simulink model "SistemaLabo_2023a"  (R2024b)
settings: Solver=VariableStepAuto  StartTime=0.0  StopTime=100  MaxStep=1e-2  RelTol=1e-3
libraries: slident x1
settings Model: Creator=david
settings DebuggingCC: UnconnectedInputMsg=warning  UnconnectedOutputMsg=warning  UnconnectedLineMsg=warning
settings ModelReferenceCC: EnableRefExpFcnMdlSchedulingChecks=on
settings RTWCC: GPUComputeCapability=3.5  DLArmComputeVersion=19.05

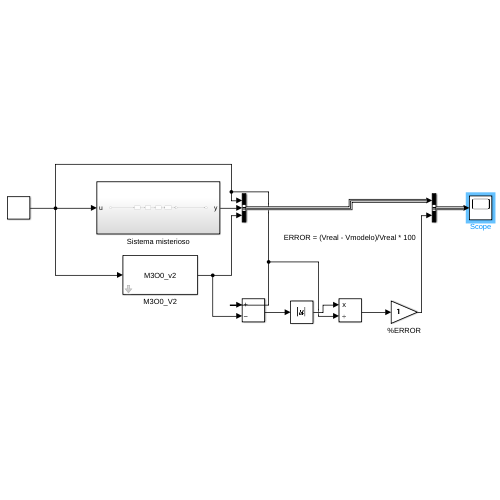
[thumbnail: Simulink's stored preview of the top-level diagram]
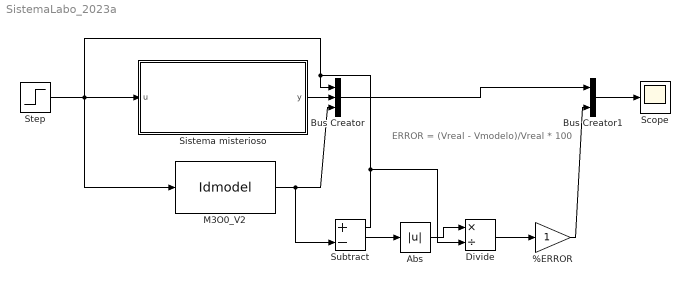
== system SistemaLabo_2023a ==
  note: ERROR = (Vreal - Vmodelo)/Vreal * 100
  %ERROR : Gain
  Abs : Abs  SaturateOnIntegerOverflow=off
  Bus Creator : BusCreator  Inputs=3
  Bus Creator1 : BusCreator  Inputs=2
  Divide : Product  Inputs=*/
  M3O0_V2 : slident/Models/Idmodel  sys=M3O0_v2  IC=0  noi=on  seed=[]
  Scope : Scope
  Sistema misterioso : Subsystem
  Step : Step  SampleTime=0
  Subtract : Sum  Inputs=+-
  wires:
  Step/1 -> Divide/2, Subtract/1, Bus Creator/1, M3O0_V2/1, Sistema misterioso/1(u)
  Sistema misterioso/1(y) -> Bus Creator/2
  M3O0_V2/1 -> Subtract/2, Bus Creator/3
  Subtract/1 -> Abs/1
  Abs/1 -> Divide/1
  Divide/1 -> %ERROR/1
  %ERROR/1 -> Bus Creator1/2
  Bus Creator/1 -> Bus Creator1/1
  Bus Creator1/1 -> Scope/1

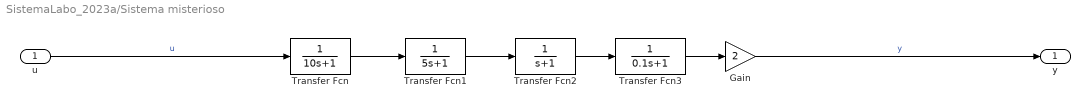
== system SistemaLabo_2023a/Sistema misterioso ==
  u : Inport
  Gain : Gain  Gain=2
  Transfer Fcn : TransferFcn  Denominator=[10 1]
  Transfer Fcn1 : TransferFcn  Denominator=[5 1]
  Transfer Fcn2 : TransferFcn  Denominator=[1 1]
  Transfer Fcn3 : TransferFcn  Denominator=[0.1 1]
  y : Outport
  wires:
  Transfer Fcn3/1 -> Gain/1
  u/1 -> Transfer Fcn/1  "u"
  Transfer Fcn2/1 -> Transfer Fcn3/1
  Transfer Fcn/1 -> Transfer Fcn1/1
  Transfer Fcn1/1 -> Transfer Fcn2/1
  Gain/1 -> y/1  "y"
